simulink model "gm_HDLLDPCDecoder"  (R2024a)
settings: Solver=FixedStepDiscrete  StartTime=0.0  StopTime=300/fs  RelTol=1e-3
undefined symbols (not defined in the file or in its folder): fs
libraries: whdledac x1, HDL_ieee_8021513 x1
settings Model: Creator=cotti  LastModifiedBy=cotti
settings OptimizationCC: BlockReduction=off  ConditionallyExecuteInputs=off  DefaultParameterBehavior=Inlined  InheritOutputTypeSmallerThanSingle=on
settings DebuggingCC: AlgebraicLoopMsg=error  ArtificialAlgebraicLoopMsg=error  InheritedTsInSrcMsg=none  SingleTaskRateTransMsg=error  UnconnectedInputMsg=warning  UnconnectedOutputMsg=warning  UnconnectedLineMsg=warning
settings HardwareCC: ProdBitPerPointer=32  ProdBitPerSizeT=32  ProdBitPerPtrDiffT=32  ProdLargestAtomicFloat=None  ProdIntDivRoundTo=Undefined  ProdEndianess=Unspecified  ProdWordSize=32  ProdHWDeviceType=ASIC/FPGA->ASIC/FPGA  TargetBitPerLong=64  TargetBitPerPointer=64  TargetBitPerSizeT=64  TargetBitPerPtrDiffT=64  TargetLongLongMode=on  TargetIntDivRoundTo=Zero  TargetEndianess=LittleEndian  TargetWordSize=64  TargetHWDeviceType=Custom Processor->MATLAB Host Computer  ProdEqTarget=off

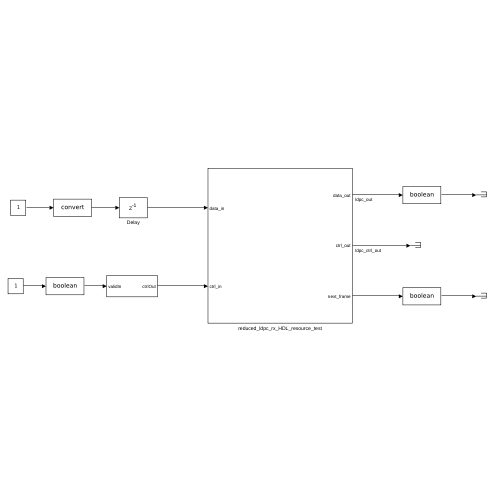
[thumbnail: Simulink's stored preview of the top-level diagram]
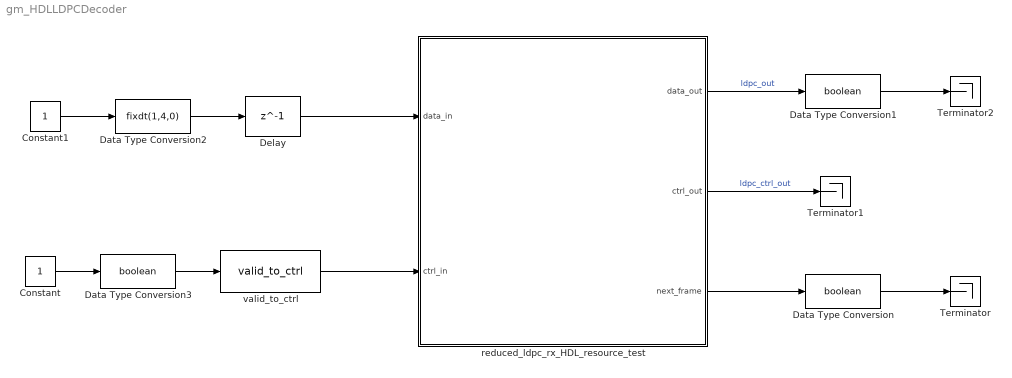
== system gm_HDLLDPCDecoder ==
  Constant : Constant  SampleTime=1/fs
  Constant1 : Constant  SampleTime=1/fs
  Data Type Conversion : DataTypeConversion  OutDataTypeStr=boolean  SaturateOnIntegerOverflow=off  RndMeth=Floor
  Data Type Conversion1 : DataTypeConversion  OutDataTypeStr=boolean  SaturateOnIntegerOverflow=off  RndMeth=Floor
  Data Type Conversion2 : DataTypeConversion  OutDataTypeStr=fixdt(1,4,0)  SaturateOnIntegerOverflow=off  RndMeth=Floor
  Data Type Conversion3 : DataTypeConversion  OutDataTypeStr=boolean  SaturateOnIntegerOverflow=off  RndMeth=Floor
  Delay : Delay  DelayLength=1  InitialCondition=0  UseCircularBuffer=on
  Terminator : Terminator
  Terminator1 : Terminator
  Terminator2 : Terminator
  reduced_ldpc_rx_HDL_resource_test : Subsystem
  valid_to_ctrl : HDL_ieee_8021513/valid_to_ctrl  SystemSampleTime=-1  VariantActivationTime=update diagram  AllowFlexibleInterface=on  Latency=0  AutoFrameSizeCalculation=off
      settings: SourceProductName=HDL IEEE 8021513
  wires:
  Constant1/1 -> Data Type Conversion2/1
  Data Type Conversion3/1 -> valid_to_ctrl/1
  Constant/1 -> Data Type Conversion3/1
  Delay/1 -> reduced_ldpc_rx_HDL_resource_test/1(data_in)
  valid_to_ctrl/1 -> reduced_ldpc_rx_HDL_resource_test/2(ctrl_in)
  Data Type Conversion2/1 -> Delay/1
  Data Type Conversion1/1 -> Terminator2/1
  reduced_ldpc_rx_HDL_resource_test/1(data_out) -> Data Type Conversion1/1  "ldpc_out"
  reduced_ldpc_rx_HDL_resource_test/2(ctrl_out) -> Terminator1/1  "ldpc_ctrl_out"
  Data Type Conversion/1 -> Terminator/1
  reduced_ldpc_rx_HDL_resource_test/3(next_frame) -> Data Type Conversion/1

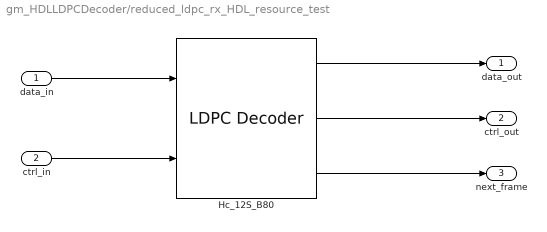
== system gm_HDLLDPCDecoder/reduced_ldpc_rx_HDL_resource_test ==
  data_in : Inport
  ctrl_in : Inport  Port=2
  Hc_12S_B80 : whdledac/LDPC Decoder  ParityCheckMatrix=Hc_12S  BlockSize=80  Algorithm=Min-sum  ScalingFactor=0.75  Termination=Max  SpecifyInputs=Property  NumIterations=4  MaxNumIterations=8  ParityCheckStatus=off  SimulateUsing=Code generation
  data_out : Outport
  ctrl_out : Outport  Port=2
  next_frame : Outport  Port=3  VectorParamsAs1DForOutWhenUnconnected=off
  wires:
  Hc_12S_B80/1 -> data_out/1
  Hc_12S_B80/2 -> ctrl_out/1
  data_in/1 -> Hc_12S_B80/1
  ctrl_in/1 -> Hc_12S_B80/2
  Hc_12S_B80/3 -> next_frame/1
